simulink model "Control_realimentacion_del_estado"  (R2017b)
settings: Solver=FixedStepAuto  StartTime=0.0  StopTime=inf  RelTol=1e-3  EnableMultiTasking=on
InitFcn:
  | TuneGain = 1
undefined symbols (not defined in the file): act, armar, gas, kk1, kk2
libraries: simulink x3, pixhawk_slib_sensors_actuators x3, dspfdesign x2
Description:
  | PX4 PSP Demo Model - parameter tune model
  | 
  | tuning parameters in external mode example
settings Model: SimulationMode=external  ParamWorkspaceSource=ReferencedWorkspace  ExtModeBatchMode=on  TunableVars=act,armar,gas,kk1,kk2,kk3,pp,pi,pd  TunableVarsStorageClass=Auto,Auto,Auto,Auto,Auto,Auto,Auto,Auto,Auto  TunableVarsTypeQualifier=,,,,,,,,  Creator=skuznick  LastModifiedBy=CPOH
settings DataIOCC: LimitDataPoints=on  SaveFormat=Array  SignalLoggingSaveFormat=ModelDataLogs
settings OptimizationCC: DefaultParameterBehavior=Inlined  LifeSpan=1  MaxStackSize=64
settings DebuggingCC: SolverPrmCheckMsg=warning  MultiTaskDSMMsg=warning  MultiTaskCondExecSysMsg=none  AllowSymbolicDim=off  SFUnexpectedBacktrackingDiag=warning  SFNoUnconditionalDefaultTransitionDiag=warning  SFExecutionAtInitializationDiag=none
settings HardwareCC: ProdBitPerPointer=32  ProdBitPerSizeT=32  ProdBitPerPtrDiffT=32  ProdLargestAtomicInteger=Long  ProdLargestAtomicFloat=Double  ProdIntDivRoundTo=Undefined  ProdWordSize=32  ProdHWDeviceType=ARM Compatible->ARM Cortex
settings ModelReferenceCC: PropagateSignalLabelsOutOfModel=off
settings SFSimCC: MATLABDynamicMemAlloc=off
settings RTWCC: SystemTargetFile=ert.tlc  HardwareBoard=Pixhawk PX4  TLCOptions=-aInlineSetEventsForThisBaseRateFcn=TLC_FALSE -aSuppressMultiTaskScheduler=TLC_FALSE -aRateBasedStepFcn=0  TemplateMakefile=ert_default_tmf  GenerateReport=on  Toolchain=Pixhawk Toolchain  IncludeHyperlinkInReport=on  LaunchReport=on  GenerateTraceInfo=on  GenerateTraceReport=on  GenerateTraceReportSl=on  GenerateTraceReportSf=on  GenerateTraceReportEml=on  GenerateCodeMetricsReport=on
settings CodeAppCC: IgnoreCustomStorageClasses=off  StateflowObjectComments=on
settings ERTTargetCC: MultiwordLength=2048  ExtMode=on  ExtModeTransport=1  ExtModeStaticAllocSize=10000  ExtModeMexFile=ext_serial_win32_comm  ExtModeMexArgs=1 4 115200  ERTCustomFileTemplate=px4_codertarget_file_process.tlc  ConvertIfToSwitch=off  SuppressUnreachableDefaultCases=off
settings ConfigComp: CovMetricSettings=dw  CovHtmlReporting=on  CovSaveCumulativeToWorkspaceVar=on  CovSaveSingleToWorkspaceVar=on  CovExternalEMLEnable=off  CovSFcnEnable=off

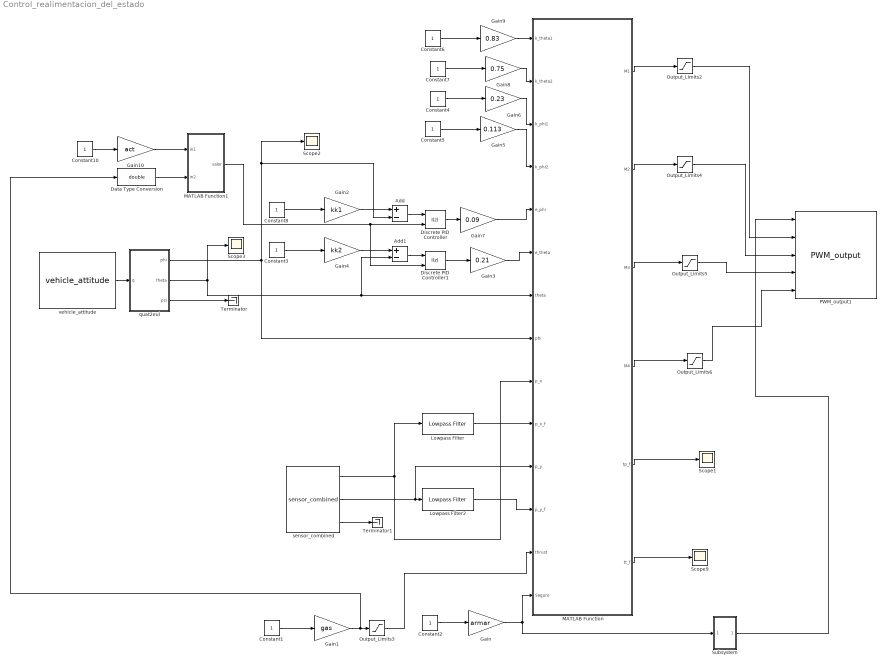
== system Control_realimentacion_del_estado ==
  Add : Sum  Inputs=+-
  Add1 : Sum  Inputs=+-
  Constant{1..8,10} (9 alike) : Constant  OutDataTypeStr=single
  Data Type Conversion : DataTypeConversion  OutDataTypeStr=double
  Discrete PID Controller : simulink/Continuous/PID Controller  Controller=I  TimeDomain=Discrete-time  SampleTime=-1  IntegratorMethod=Forward Euler  FilterMethod=Forward Euler  Form=Parallel  UseFilter=on  ControllerParametersSource=internal  P=1  I=1  D=0  N=100  InitialConditionSource=internal  InitialConditionForIntegrator=0  InitialConditionForFilter=0  ExternalReset=level  LimitOutput=off  UpperSaturationLimit=inf  LowerSaturationLimit=-inf  LinearizeAsGain=off  AntiWindupMode=none  Kb=1  TrackingMode=off  Kt=1  PParamMin=[]  PParamMax=[]  IParamMin=[]  IParamMax=[]  DParamMin=[]  DParamMax=[]  NParamMin=[]  NParamMax=[]  KbParamMin=[]  KbParamMax=[]  KtParamMin=[]  KtParamMax=[]  POutMin=[]  POutMax=[]  IOutMin=[]  IOutMax=[]  DOutMin=[]  DOutMax=[]  NOutMin=[]  NOutMax=[]  KbOutMin=[]  KbOutMax=[]  KtOutMin=[]  KtOutMax=[]  IntegratorOutMin=[]  IntegratorOutMax=[]  FilterOutMin=[]  FilterOutMax=[]  SumOutMin=[]  SumOutMax=[]  SumI1OutMin=[]  SumI1OutMax=[]  SumI2OutMin=[]  SumI2OutMax=[]  SumI3OutMin=[]  SumI3OutMax=[]  SumDOutMin=[]  SumDOutMax=[]  SaturationOutMin=[]  SaturationOutMax=[]  IntegratorContinuousStateAttributes=''  IntegratorStateMustResolveToSignalObject=off  IntegratorRTWStateStorageClass=Auto  FilterContinuousStateAttributes=''  FilterStateMustResolveToSignalObject=off  FilterRTWStateStorageClass=Auto  DifferentiatorICPrevScaledInput=0  DifferentiatorOutMin=[]  DifferentiatorOutMax=[]  InitialConditionSetting=State (most efficient)  FilterDiffOutCoefMin=[]  FilterDiffOutCoefMax=[]  SumDenOutMin=[]  SumDenOutMax=[]  SumNumOutMin=[]  SumNumOutMax=[]  ReciprocalOutMin=[]  ReciprocalOutMax=[]  DivideOutMin=[]  DivideOutMax=[]  TunerSelectOption=Transfer Function Based (PID Tuner App)
  Discrete PID Controller1 : simulink/Continuous/PID Controller  Controller=I  TimeDomain=Discrete-time  SampleTime=-1  IntegratorMethod=Forward Euler  FilterMethod=Forward Euler  Form=Parallel  UseFilter=on  ControllerParametersSource=internal  P=1  I=1  D=0  N=100  InitialConditionSource=internal  InitialConditionForIntegrator=0  InitialConditionForFilter=0  ExternalReset=level  LimitOutput=off  UpperSaturationLimit=inf  LowerSaturationLimit=-inf  LinearizeAsGain=off  AntiWindupMode=none  Kb=1  TrackingMode=off  Kt=1  PParamMin=[]  PParamMax=[]  IParamMin=[]  IParamMax=[]  DParamMin=[]  DParamMax=[]  NParamMin=[]  NParamMax=[]  KbParamMin=[]  KbParamMax=[]  KtParamMin=[]  KtParamMax=[]  POutMin=[]  POutMax=[]  IOutMin=[]  IOutMax=[]  DOutMin=[]  DOutMax=[]  NOutMin=[]  NOutMax=[]  KbOutMin=[]  KbOutMax=[]  KtOutMin=[]  KtOutMax=[]  IntegratorOutMin=[]  IntegratorOutMax=[]  FilterOutMin=[]  FilterOutMax=[]  SumOutMin=[]  SumOutMax=[]  SumI1OutMin=[]  SumI1OutMax=[]  SumI2OutMin=[]  SumI2OutMax=[]  SumI3OutMin=[]  SumI3OutMax=[]  SumDOutMin=[]  SumDOutMax=[]  SaturationOutMin=[]  SaturationOutMax=[]  IntegratorContinuousStateAttributes=''  IntegratorStateMustResolveToSignalObject=off  IntegratorRTWStateStorageClass=Auto  FilterContinuousStateAttributes=''  FilterStateMustResolveToSignalObject=off  FilterRTWStateStorageClass=Auto  DifferentiatorICPrevScaledInput=0  DifferentiatorOutMin=[]  DifferentiatorOutMax=[]  InitialConditionSetting=State (most efficient)  FilterDiffOutCoefMin=[]  FilterDiffOutCoefMax=[]  SumDenOutMin=[]  SumDenOutMax=[]  SumNumOutMin=[]  SumNumOutMax=[]  ReciprocalOutMin=[]  ReciprocalOutMax=[]  DivideOutMin=[]  DivideOutMax=[]  TunerSelectOption=Transfer Function Based (PID Tuner App)
  Gain : Gain  Gain=armar
  Gain1 : Gain  Gain=gas
  Gain10 : Gain  Gain=act
  Gain2 : Gain  Gain=kk1
  Gain3 : Gain  Gain=0.21
  Gain4 : Gain  Gain=kk2
  Gain5 : Gain  Gain=0.113
  Gain6 : Gain  Gain=0.23
  Gain7 : Gain  Gain=0.09
  Gain8 : Gain  Gain=0.75
  Gain9 : Gain  Gain=0.83
  Lowpass Filter : dspfdesign/Lowpass Filter  FilterType=FIR  DesignForMinimumOrder=off  FilterOrder=3  PassbandFrequency=8e3  StopbandFrequency=2e3  PassbandRipple=0.5  StopbandAttenuation=110  InheritSampleRate=off  SampleRate=44100  SimulateUsing=Interpreted execution  roundingMode=Floor  coeffsDataTypeStr=fixdt(1,16)
  Lowpass Filter2 : dspfdesign/Lowpass Filter  FilterType=FIR  DesignForMinimumOrder=off  FilterOrder=3  PassbandFrequency=8e3  StopbandFrequency=2e3  PassbandRipple=0.5  StopbandAttenuation=110  InheritSampleRate=off  SampleRate=44100  SimulateUsing=Interpreted execution  roundingMode=Floor  coeffsDataTypeStr=fixdt(1,16)
  MATLAB Function : MATLAB Function  TreatAsAtomicUnit=on
  MATLAB Function1 : MATLAB Function  TreatAsAtomicUnit=on
  Output_Limits{2,4..6} (4 alike) : Saturate  UpperLimit=1500  LowerLimit=1000
  Output_Limits3 : Saturate  UpperLimit=40  LowerLimit=0
  PWM_output1 : pixhawk_slib_sensors_actuators/PWM_output  pub_outputs=on  pwm_rate=400Hz  show_pwm1=on  show_pwm5=off  show_pwm2=on  show_pwm6=off  show_pwm3=on  show_pwm7=off  show_pwm4=on  show_pwm8=off
      settings: SourceProductName=Pixhawk Target Blocks
  Scope{1..3,9} (4 alike) : Scope
  Subsystem : Subsystem
  Terminator : Terminator
  Terminator1 : Terminator
  quat2eul : MATLAB Function  TreatAsAtomicUnit=on
  sensor_combined : pixhawk_slib_sensors_actuators/sensor_combined  sampletime=1/250  show_mag=off  show_acc=off  show_gyro=on  show_baro=off  show_ts=off
      settings: SourceProductName=Pixhawk Target Blocks
  vehicle_attitude : pixhawk_slib_sensors_actuators/vehicle_attitude  sampletime=0.004  show_r=off  show_p=off  show_y=off  show_q=on  show_ts=off
      settings: SourceProductName=Pixhawk Target Blocks
  wires:
  Output_Limits5/1 -> PWM_output1/4
  Output_Limits4/1 -> PWM_output1/3
  Gain/1 -> Subsystem/1(In1), MATLAB Function/14(Seguro)
  Output_Limits6/1 -> PWM_output1/5
  MATLAB Function/2(M2) -> Output_Limits4/1
  MATLAB Function/4(M4) -> Output_Limits6/1
  MATLAB Function/1(M1) -> Output_Limits2/1
  MATLAB Function/3(M3) -> Output_Limits5/1
  Output_Limits2/1 -> PWM_output1/2
  Constant1/1 -> Gain1/1
  Output_Limits3/1 -> MATLAB Function/13(thrust)
  quat2eul/1(phi) -> MATLAB Function/8(phi), Scope2/1, Add/2
  sensor_combined/2 -> MATLAB Function/11(p_y), Lowpass Filter2/1
  sensor_combined/1 -> Lowpass Filter/1, MATLAB Function/9(p_x)
  vehicle_attitude/1 -> quat2eul/1(q)
  Constant2/1 -> Gain/1
  Constant8/1 -> Gain2/1
  Gain2/1 -> Add/1
  Add/1 -> Discrete PID Controller/1
  Discrete PID Controller/1 -> Gain7/1
  Gain7/1 -> MATLAB Function/5(e_phi)
  Gain3/1 -> MATLAB Function/6(e_theta)
  Discrete PID Controller1/1 -> Gain3/1
  Add1/1 -> Discrete PID Controller1/1
  quat2eul/2(theta) -> Add1/2, MATLAB Function/7(theta), Scope3/1
  Constant3/1 -> Gain4/1
  Gain4/1 -> Add1/1
  Subsystem/1(Out1) -> PWM_output1/1
  Constant4/1 -> Gain6/1
  Constant5/1 -> Gain5/1
  Constant7/1 -> Gain8/1
  Constant6/1 -> Gain9/1
  Gain9/1 -> MATLAB Function/1(k_theta1)
  Gain8/1 -> MATLAB Function/2(k_theta2)
  Gain6/1 -> MATLAB Function/3(k_phi1)
  Gain5/1 -> MATLAB Function/4(k_phi2)
  Gain1/1 -> Data Type Conversion/1, Output_Limits3/1
  MATLAB Function1/1(valor) -> Discrete PID Controller1/2, Discrete PID Controller/2
  Gain10/1 -> MATLAB Function1/1(in1)
  Data Type Conversion/1 -> MATLAB Function1/2(in2)
  Constant10/1 -> Gain10/1
  MATLAB Function/5(tp_f) -> Scope1/1
  MATLAB Function/6(tt_f) -> Scope9/1
  Lowpass Filter/1 -> MATLAB Function/10(p_x_f)
  Lowpass Filter2/1 -> MATLAB Function/12(p_y_f)
  quat2eul/3(psi) -> Terminator/1
  sensor_combined/3 -> Terminator1/1

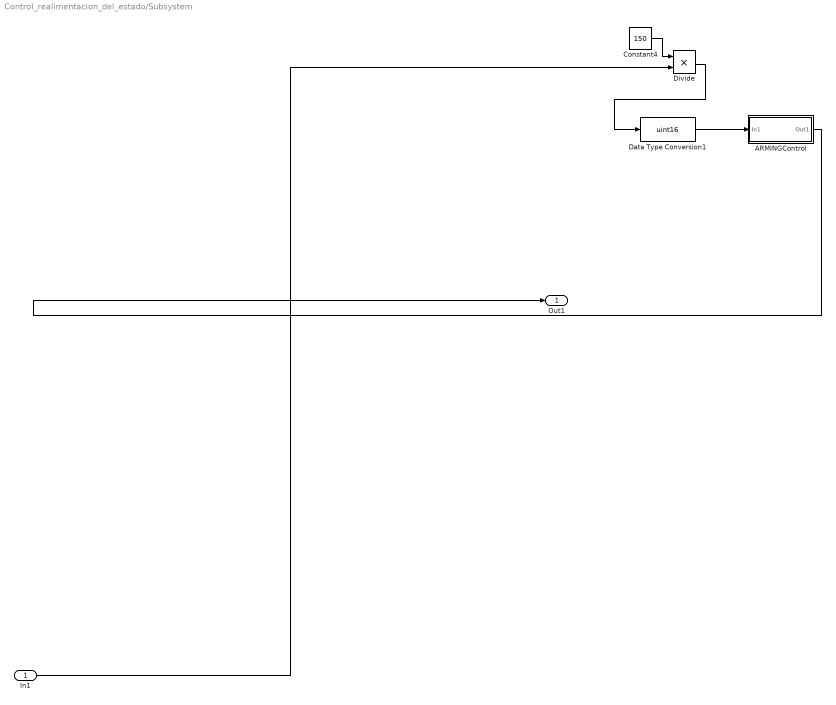
== system Control_realimentacion_del_estado/Subsystem ==
  In1 : Inport
  ARMINGControl : Subsystem
  Constant4 : Constant  Value=150  OutDataTypeStr=uint16
  Data Type Conversion1 : DataTypeConversion  OutDataTypeStr=uint16
  Divide : Product  Inputs=**
  Out1 : Outport
  wires:
  In1/1 -> Divide/2
  Constant4/1 -> Divide/1
  Data Type Conversion1/1 -> ARMINGControl/1(In1)
  ARMINGControl/1(Out1) -> Out1/1
  Divide/1 -> Data Type Conversion1/1

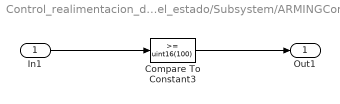
== system Control_realimentacion_del_estado/Subsystem/ARMINGControl ==
  In1 : Inport
  Compare To Constant3 : simulink/Logic and Bit Operations/Compare To Constant  relop=>=  const=uint16(100)  OutDataTypeStr=boolean
  Out1 : Outport
  wires:
  Compare To Constant3/1 -> Out1/1
  In1/1 -> Compare To Constant3/1

== matlab function Control_realimentacion_del_estado/MATLAB Function ==
  data: k_theta1 input; k_theta2 input; k_phi1 input; k_phi2 input; e_phi input; e_theta input; theta input; M1 output; phi input; p_x input; p_x_f input; p_y input; p_y_f input; M2 output; M3 output; M4 output; thrust input; Seguro input; tp_f output; tt_f output
function [M1,M2,M3,M4,tp_f,tt_f] = fcn(k_theta1,k_theta2,k_phi1,k_phi2,e_phi,e_theta,theta,phi,p_x, p_x_f,p_y,p_y_f,thrust,Seguro)




db=0.0912; %Diagonal de motor al cento= 129 mm
nb=0.25; %4 brazos = 1/4  %Fuerza entre 4

%Coeficientes funcion PWM-thrust motor a*x^2+b*x+c
a=0.0452;
b=21.649;
%c=2.86;
c=0;

pitch=0;
roll=0;
yaw=0;

ke_psi=0;
%e_psi=0;


%pitch=(k_theta1*theta+k_theta2*p_y+e_theta);
pitch=(k_theta1*theta+k_theta2*p_y-e_theta);
roll=(k_phi1*phi+k_phi2*p_x-e_phi);
yaw=(k_psi1*psi+k_psi2*p_z-e_psi);

pitch_f=(k_theta1*theta+k_theta2*p_y_f-e_theta);
roll_f=(k_phi1*phi+k_phi2*p_x_f-e_phi);
%yaw_f=(k_psi1*psi+k_psi2*p_z_f-e_psi);


tp=roll;
tt=pitch;
tpp=yaw;

tp_f=roll_f;
tt_f=pitch_f;

roll=tp_f;
pitch=tt_f;
%tpp_f=yaw_f;
%Torque entre 4 motores (entre 4, entre 2 =1/8)

pitch=pitch*nb/db; 
roll=roll*nb/db;
yaw=yaw*nb/db;

pitch=a*pitch^2+b*pitch+c;
roll=a*roll^2+b*roll+c;
yaw=a*yaw^2+b*yaw+c;

pitch=-pitch;
roll=-roll;
yaw=-yaw;
%inhabilitar yaw

%roll=0;
yaw=0;
%pitch=0;

% MIXER MOTORES -------------------------------------------------
idle_PWM = uint16(1000);

M1=uint16((roll+pitch-yaw+thrust)*10)+idle_PWM;
M2=uint16((-roll+pitch+yaw+thrust)*10)+idle_PWM;
M3=uint16((-roll-pitch-yaw+thrust)*10)+idle_PWM;
M4=uint16((roll-pitch+yaw+thrust)*10)+idle_PWM;



if Seguro==0
   M1=idle_PWM;
   M2=idle_PWM;
   M3=idle_PWM;
   M4=idle_PWM;
   
end

== matlab function Control_realimentacion_del_estado/MATLAB Function1 ==
  data: in1 input; valor output; in2 input
function valor  = fcn(in1,in2)
h=in2;

if in1>0
   h=0; 
end

valor=h;

== matlab function Control_realimentacion_del_estado/quat2eul ==
  data: q input; phi output; theta output; psi output
function [phi,theta,psi] = quat2eul(q)
% Conversion from Quaternion to Euler angles based on the PX4 Firmware
% v1.6.5 release.
% 
% Quaternion -> DCM -> Euler Angles
% INPUT:
%   q: Quaternion vector of the format: (a + bi + cj + dk)
% OUTPUT:
%   [phi,theta,psi]: Euler angles in radians.
% 
 
    a = q(1);
    b = q(2);
    c = q(3);
    d = q(4);

    aSq = a*a;
    bSq = b*b;
    cSq = c*c;
    dSq = d*d;

    d_pi2 = pi/2;

    % quaternion_to_dcm
    dcm00 = aSq + bSq - cSq - dSq;
    % dcm01 = 2*(b*c - a*d);
    dcm02 = 2*(a*c + b*d);
    dcm10 = 2*(b*c + a*d);
    % dcm11 = aSq - bSq + cSq - dSq;
    dcm12 = 2*(c*d - a*b);
    dcm20 = 2*(b*d - a*c);
    dcm21 = 2*(a*b + c*d);
    dcm22 = aSq - bSq - cSq + dSq;

    % dcm_to_euler
    theta = asin(-dcm20);
    if abs(theta - d_pi2) < 1.0e-3
        phi = single(0.0);
        psi = atan2(dcm12, dcm02);
    elseif abs(theta + d_pi2) < 1.0e-3
        phi = single(0.0);
        psi = atan2(-dcm12, -dcm02);
    else
        phi = atan2(dcm21, dcm22);
        psi = atan2(dcm10, dcm00);
    end

end
